simulink model "Part5"  (R2021a)
settings: Solver=VariableStepAuto  StartTime=0.0  StopTime=10.0  RelTol=1e-3
undefined symbols (not defined in the file): A, B, C, k, x0
settings Model: Creator=ASUS  LastModifiedBy=ASUS

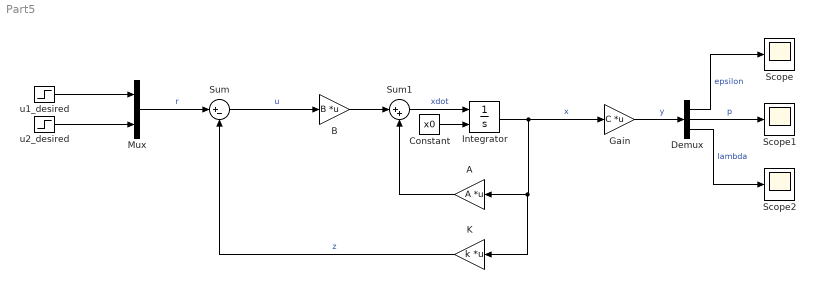
== system Part5 ==
  A : Gain  Gain=A  Multiplication=Matrix(K*u)
  B : Gain  Gain=B  Multiplication=Matrix(K*u)
  Constant : Constant  Value=x0
  Demux : Demux  Outputs=3
  Gain : Gain  Gain=C  Multiplication=Matrix(K*u)
  Integrator : Integrator  InitialConditionSource=external
  K : Gain  Gain=k  Multiplication=Matrix(K*u)
  Mux : Mux  Inputs=2
  Scope : Scope
  Scope1 : Scope
  Scope2 : Scope
  Sum : Sum  Inputs=|+-
  Sum1 : Sum  Inputs=|++
  u1_desired : Step  Time=0  After=0  SampleTime=0
  u2_desired : Step  Time=0  After=0  SampleTime=0
  wires:
  u1_desired/1 -> Mux/1
  u2_desired/1 -> Mux/2
  Mux/1 -> Sum/1  "r"
  K/1 -> Sum/2  "z"
  Sum/1 -> B/1  "u"
  B/1 -> Sum1/1
  A/1 -> Sum1/2
  Sum1/1 -> Integrator/1  "xdot"
  Integrator/1 -> K/1, A/1, Gain/1  "x"
  Gain/1 -> Demux/1  "y"
  Demux/1 -> Scope/1  "epsilon"
  Demux/2 -> Scope1/1  "p"
  Demux/3 -> Scope2/1  "lambda"
  Constant/1 -> Integrator/2
